simulink model "harness"  (Simulink 7.0)
settings: Solver=ode23  StartTime=0.0  StopTime=20  FixedStep=0.01  RelTol=1e-3
InitFcn:
  | init_simulation
StopFcn:
  | post_simulation
values from neighbouring files (symbols this model uses):
  A = pi*R^2    (= 0.0506707479097)    [constants.m]
  accel_noise = noise_on*.01^2    [constants.m]
  Alpha = pi/180*[-85:5:85]    [constants.m]
  att_noise = noise_on*(.25*pi/180)^2    [constants.m]
  att_ref = [0.2 0.2 0 0 0 0]'    [run_simulation.m]
  att_traj_on = 0    [set_scenario.m]
  b = 0.1    [constants.m]
  const_wind = [1 1 0]    [run_simulation.m]
  g = [0 0 9.8]'    [constants.m]
  gyro_noise = noise_on*.01^2    [constants.m]
  J = [Jxx 0 0 ... (first row only)    [constants.m]
  K_a1s = .009    (= 0.009)    [constants.m]
  K_attitude = [  0   kp_p   kp_y     0    kd_p   kd_y ... (first row only)    [run_simulation.m]
  K_beta = 0.23    [constants.m]
  K_dz = 0.7    [run_simulation.m]
  K_flap = 4*(K_beta + T_nom*dz)*K_a1s/(2*dx)    (= 0.0320793572835)    [constants.m]
  K_pz = .37    (= 0.37)    [run_simulation.m]
  K_torque = 0.47    [constants.m]
  M = 1.8263    [constants.m]
  motor_noise = noise_on*(9.8/4*.05)^2    [constants.m]
  plant_int_period = t_s / tau_motor    (= 0.00131578947368)    [constants.m]
  pos_noise = noise_on*0.02^2    [constants.m]
  r1 = [dx 0 -dz]'    [constants.m]
  r2 = [0 dx -dz]'    [constants.m]
  r3 = [-dx 0 -dz]'    [constants.m]
  r4 = [0 -dx -dz]'    [constants.m]
  R_90 = [0 -1 0 ... (first row only)    [constants.m]
  rho = 1.2    [constants.m]
  select = 0    [run_simulation.m]
  T_nom = M*9.8/4    (= 4.474435)    [constants.m]
  t_s = 1/76    (= 0.0131578947368)    [constants.m]
  tau_motor = 10    [constants.m]
  thrust_max = 9.8 * 1    (= 9.8)    [constants.m]
  thrust_min = 0    [constants.m]
  v_min = 1e-3    (= 0.001)    [constants.m]
  vel_noise = noise_on*0.05^2    [constants.m]
  Vh = sqrt(T/(2*rho*A))    [constants.m]
  Vinf = [0:0.5:6]    [constants.m]
  w_seed = 0    [run_simulation.m]
  wind = 3    [run_simulation.m]
  wind_clip = wind_max    (= 10)    [run_simulation.m]
  wind_duration = 5    [run_simulation.m]
  wind_max = 10    [run_simulation.m]
  wind_start = 3    [run_simulation.m]
  wind_var = (wind_max / 10)^2    (= 1)    [run_simulation.m]
  wind_vector = [1 0 0]'    [run_simulation.m]
  zd_ref = 0    [run_simulation.m]
undefined symbols (not defined in the file or in its folder): DiscIntNeverNeededParam, ToverTh
libraries: simulink x20
(part 2 of 3)

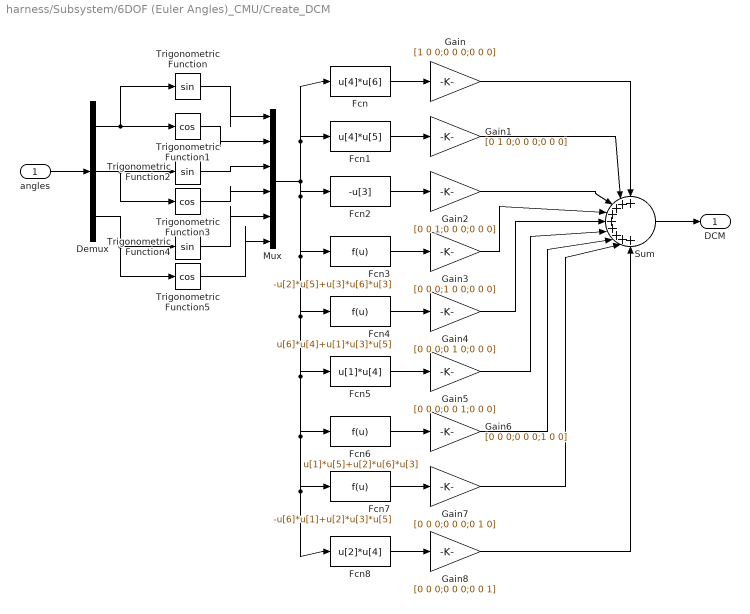
== system harness/Subsystem/6DOF (Euler Angles)_CMU/Create_DCM ==
  angles : Inport  OutDataType=sfix(16)  OutScaling=2^0
  Demux : Demux  Outputs=3
  Fcn : Fcn  Expr=u[4]*u[6]
  Fcn1 : Fcn  Expr=u[4]*u[5]
  Fcn2 : Fcn  Expr=-u[3]
  Fcn3 : Fcn  Expr=-u[2]*u[5]+u[3]*u[6]*u[3]
  Fcn4 : Fcn  Expr=u[6]*u[4]+u[1]*u[3]*u[5]
  Fcn5 : Fcn  Expr=u[1]*u[4]
  Fcn6 : Fcn  Expr=u[1]*u[5]+u[2]*u[6]*u[3]
  Fcn7 : Fcn  Expr=-u[6]*u[1]+u[2]*u[3]*u[5]
  Fcn8 : Fcn  Expr=u[2]*u[4]
  Gain : Gain  Gain=[1 0 0;0 0 0;0 0 0]  ParameterDataType=sfix(16)  ParameterScaling=2^0  OutDataType=sfix(16)  OutScaling=2^0
  Gain1 : Gain  Gain=[0 1 0;0 0 0;0 0 0]  ParameterDataType=sfix(16)  ParameterScaling=2^0  OutDataType=sfix(16)  OutScaling=2^0
  Gain2 : Gain  Gain=[0 0 1;0 0 0;0 0 0]  ParameterDataType=sfix(16)  ParameterScaling=2^0  OutDataType=sfix(16)  OutScaling=2^0
  Gain3 : Gain  Gain=[0 0 0;1 0 0;0 0 0]  ParameterDataType=sfix(16)  ParameterScaling=2^0  OutDataType=sfix(16)  OutScaling=2^0
  Gain4 : Gain  Gain=[0 0 0;0 1 0;0 0 0]  ParameterDataType=sfix(16)  ParameterScaling=2^0  OutDataType=sfix(16)  OutScaling=2^0
  Gain5 : Gain  Gain=[0 0 0;0 0 1;0 0 0]  ParameterDataType=sfix(16)  ParameterScaling=2^0  OutDataType=sfix(16)  OutScaling=2^0
  Gain6 : Gain  Gain=[0 0 0;0 0 0;1 0 0]  ParameterDataType=sfix(16)  ParameterScaling=2^0  OutDataType=sfix(16)  OutScaling=2^0
  Gain7 : Gain  Gain=[0 0 0;0 0 0;0 1 0]  ParameterDataType=sfix(16)  ParameterScaling=2^0  OutDataType=sfix(16)  OutScaling=2^0
  Gain8 : Gain  Gain=[0 0 0;0 0 0;0 0 1]  ParameterDataType=sfix(16)  ParameterScaling=2^0  OutDataType=sfix(16)  OutScaling=2^0
  Mux : Mux  Inputs=6
  Sum : Sum  Inputs=+++++++++  OutDataType=sfix(16)  OutScaling=2^0
  Trigonometric Function : Trigonometry
  Trigonometric Function1 : Trigonometry  Operator=cos
  Trigonometric Function2 : Trigonometry
  Trigonometric Function3 : Trigonometry  Operator=cos
  Trigonometric Function4 : Trigonometry
  Trigonometric Function5 : Trigonometry  Operator=cos
  DCM : Outport  OutDataType=sfix(16)  OutScaling=2^0
  wires:
  Sum/1 -> DCM/1
  Gain8/1 -> Sum/9
  Fcn8/1 -> Gain8/1
  Gain7/1 -> Sum/8
  Fcn7/1 -> Gain7/1
  Gain6/1 -> Sum/7
  Fcn6/1 -> Gain6/1
  Gain5/1 -> Sum/6
  Fcn5/1 -> Gain5/1
  Gain4/1 -> Sum/5
  Fcn4/1 -> Gain4/1
  Gain3/1 -> Sum/4
  Fcn3/1 -> Gain3/1
  Gain2/1 -> Sum/3
  Fcn2/1 -> Gain2/1
  Gain1/1 -> Sum/2
  Fcn1/1 -> Gain1/1
  Gain/1 -> Sum/1
  Fcn/1 -> Gain/1
  Mux/1 -> Fcn8/1, Fcn7/1, Fcn6/1, Fcn5/1, Fcn4/1, Fcn3/1, Fcn2/1, Fcn1/1, Fcn/1
  Trigonometric Function5/1 -> Mux/6
  Trigonometric Function4/1 -> Mux/5
  Trigonometric Function3/1 -> Mux/4
  Trigonometric Function2/1 -> Mux/3
  Trigonometric Function1/1 -> Mux/2
  Trigonometric Function/1 -> Mux/1
  Demux/3 -> Trigonometric Function5/1, Trigonometric Function4/1
  Demux/2 -> Trigonometric Function3/1, Trigonometric Function2/1
  Demux/1 -> Trigonometric Function1/1, Trigonometric Function/1
  angles/1 -> Demux/1

== system harness/Subsystem/6DOF (Euler Angles)_CMU/CrossProduct(AXB) ==
  A : Inport  OutDataType=sfix(16)  OutScaling=2^0
  B : Inport  Port=2  OutDataType=sfix(16)  OutScaling=2^0
  Fcn : Fcn  Expr=u[2]*u[6]-u[3]*u[5]
  Fcn1 : Fcn  Expr=u[3]*u[4]-u[1]*u[6]
  Fcn2 : Fcn  Expr=u[1]*u[5]-u[2]*u[4]
  Mux : Mux  Inputs=2
  Mux1 : Mux  Inputs=3
  Out : Outport  OutDataType=sfix(16)  OutScaling=2^0
  wires:
  Mux1/1 -> Out/1
  Fcn2/1 -> Mux1/3
  Fcn1/1 -> Mux1/2
  Fcn/1 -> Mux1/1
  Mux/1 -> Fcn2/1, Fcn1/1, Fcn/1
  B/1 -> Mux/2
  A/1 -> Mux/1

== system harness/Subsystem/6DOF (Euler Angles)_CMU/CrossProduct(AXB)1 ==
  A : Inport  OutDataType=sfix(16)  OutScaling=2^0
  B : Inport  Port=2  OutDataType=sfix(16)  OutScaling=2^0
  Fcn : Fcn  Expr=u[2]*u[6]-u[3]*u[5]
  Fcn1 : Fcn  Expr=u[3]*u[4]-u[1]*u[6]
  Fcn2 : Fcn  Expr=u[1]*u[5]-u[2]*u[4]
  Mux : Mux  Inputs=2
  Mux1 : Mux  Inputs=3
  Out : Outport  OutDataType=sfix(16)  OutScaling=2^0
  wires:
  A/1 -> Mux/1
  B/1 -> Mux/2
  Mux/1 -> Fcn/1, Fcn1/1, Fcn2/1
  Fcn/1 -> Mux1/1
  Fcn1/1 -> Mux1/2
  Fcn2/1 -> Mux1/3
  Mux1/1 -> Out/1

== system harness/Subsystem/Aerodynamic Effects/Flapping Dynamics ==
  Vb2_hat : Inport  OutDataType=sfix(16)  OutScaling=2^0
  "Body Z " : Constant  Value=[0; 0; -1];  OutDataType=sfix(16)  OutScaling=2^0
  Constant : Constant  OutDataType=sfix(16)  OutScaling=2^0
  Constant1 : Constant  Value=1/v_min  OutDataType=sfix(16)  OutScaling=2^0
  Constant2 : Constant  Value=[0 0 0]'  OutDataType=sfix(16)  OutScaling=2^0
  Divide : Product  Inputs=*/  OutDataType=sfix(16)  OutScaling=2^-10
  Dot Product : simulink/Math Operations/Dot Product  InputSameDT=on  OutDataType=sfix(16)  OutScaling=2^-10  DoSatur=off
  Flap Angle Gain : Gain  Gain=K_a1s  ParameterDataType=sfix(16)  ParameterScaling=2^0  OutDataType=sfix(16)  OutScaling=2^0
  Gain : Gain  Gain=-1  ParameterDataType=sfix(16)  ParameterScaling=2^0  OutDataType=sfix(16)  OutScaling=2^0
  Gain1 : Gain  Gain=K_beta  ParameterDataType=sfix(16)  ParameterScaling=2^0  OutDataType=sfix(16)  OutScaling=2^0
  Gain2 : Gain  Gain=4  ParameterDataType=sfix(16)  ParameterScaling=2^0  OutDataType=sfix(16)  OutScaling=2^0
  Math Function : Math  Operator=sqrt  OutDataType=sfix(16)  OutScaling=2^0  SaturateOnIntegerOverflow=on
  Product{1..4} (4 alike) : Product  OutDataType=sfix(16)  OutScaling=2^0  RndMeth=Zero
  Sum : Sum  Inputs=|++  OutDataType=sfix(16)  OutScaling=2^0
  Switch : Switch  Threshold=v_min
  Trigonometric Function : Trigonometry
  Trigonometric Function1 : Trigonometry  Operator=cos
  flap moments : Scope
      settings: SaveName=ScopeData10
  flapping switch : Switch  Threshold=v_min
  rotate 90 degrees : Gain  Gain=R_90  Multiplication=Matrix(K*u)  ParameterDataType=sfix(16)  ParameterScaling=2^0  OutDataType=sfix(16)  OutScaling=2^0
  v : Scope
      settings: SaveName=ScopeData6
  thrust vector : Outport  OutDataType=sfix(16)  OutScaling=2^0
  rotor blade moments : Outport  Port=2  OutDataType=sfix(16)  OutScaling=2^0
  wires:
  Product4/1 -> Trigonometric Function1/1, Trigonometric Function/1, Gain1/1, v/1  "flap angle"
  Vb2_hat/1 -> Dot Product/1, Dot Product/2, Divide/1
  Dot Product/1 -> Math Function/1
  Math Function/1 -> Switch/1, Switch/2, flapping switch/2, Flap Angle Gain/1  "v"
  Trigonometric Function1/1 -> Product1/2
  Trigonometric Function/1 -> Product3/1
  Product3/1 -> Sum/2
  Gain/1 -> Product3/2
  Product1/1 -> Sum/1
  "Body Z "/1 -> Product1/1
  Sum/1 -> thrust vector/1
  Gain2/1 -> rotor blade moments/1, flap moments/1
  Switch/1 -> Divide/2
  Constant1/1 -> Switch/3
  Divide/1 -> flapping switch/1  "unit vector"
  flapping switch/1 -> Gain/1, rotate 90 degrees/1
  Constant2/1 -> flapping switch/3
  Product2/1 -> Gain2/1
  rotate 90 degrees/1 -> Product2/2
  Gain1/1 -> Product2/1
  Flap Angle Gain/1 -> Product4/2
  Constant/1 -> Product4/1

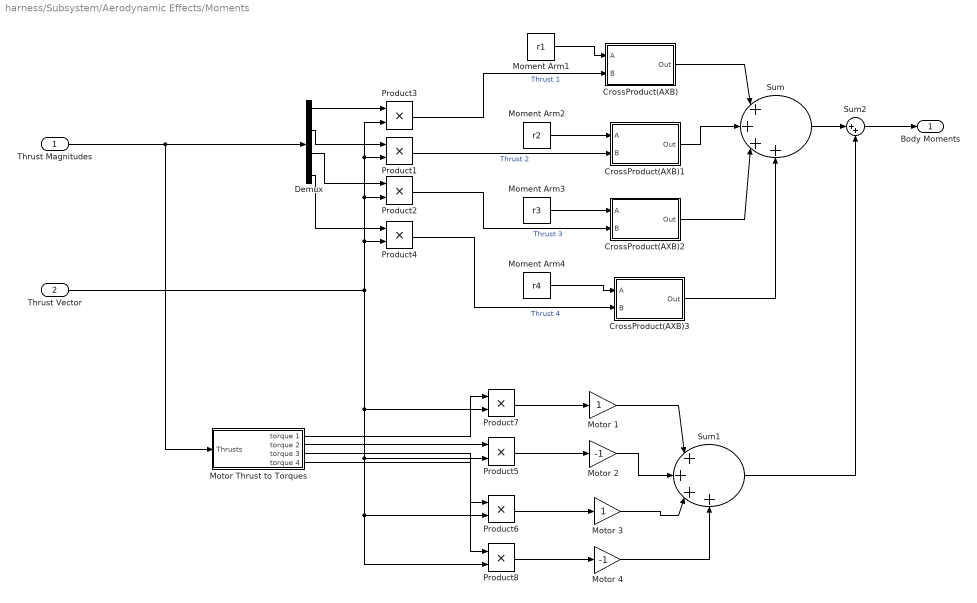
== system harness/Subsystem/Aerodynamic Effects/Moments ==
  Thrust Magnitudes : Inport  OutDataType=sfix(16)  OutScaling=2^0
  Thrust Vector : Inport  Port=2  OutDataType=sfix(16)  OutScaling=2^0
  CrossProduct(AXB) : Subsystem
  CrossProduct(AXB)1 : Subsystem
  CrossProduct(AXB)2 : Subsystem
  CrossProduct(AXB)3 : Subsystem
  Demux : Demux
  Moment Arm1 : Constant  Value=r1  OutDataType=sfix(16)  OutScaling=2^0
  Moment Arm2 : Constant  Value=r2  OutDataType=sfix(16)  OutScaling=2^0
  Moment Arm3 : Constant  Value=r3  OutDataType=sfix(16)  OutScaling=2^0
  Moment Arm4 : Constant  Value=r4  OutDataType=sfix(16)  OutScaling=2^0
  Motor 1 : Gain  ParameterDataType=sfix(16)  ParameterScaling=2^0  OutDataType=sfix(16)  OutScaling=2^0
  Motor 2 : Gain  Gain=-1  ParameterDataType=sfix(16)  ParameterScaling=2^0  OutDataType=sfix(16)  OutScaling=2^0
  Motor 3 : Gain  ParameterDataType=sfix(16)  ParameterScaling=2^0  OutDataType=sfix(16)  OutScaling=2^0
  Motor 4 : Gain  Gain=-1  ParameterDataType=sfix(16)  ParameterScaling=2^0  OutDataType=sfix(16)  OutScaling=2^0
  Motor Thrust to Torques : Subsystem
  Product{1..8} (8 alike) : Product  OutDataType=sfix(16)  OutScaling=2^0  RndMeth=Zero
  Sum : Sum  Inputs=|++++  OutDataType=sfix(16)  OutScaling=2^0
  Sum1 : Sum  Inputs=|++++  OutDataType=sfix(16)  OutScaling=2^0
  Sum2 : Sum  Inputs=|++  OutDataType=sfix(16)  OutScaling=2^0
  Body Moments : Outport  OutDataType=sfix(16)  OutScaling=2^0
  wires:
  Thrust Magnitudes/1 -> Demux/1, Motor Thrust to Torques/1(Thrusts)
  Demux/1 -> Product3/1
  Demux/2 -> Product1/1
  Demux/3 -> Product2/1
  Demux/4 -> Product4/1
  Thrust Vector/1 -> Product3/2, Product1/2, Product2/2, Product4/2, Product7/2, Product5/2, Product6/2, Product8/2
  Moment Arm1/1 -> CrossProduct(AXB)/1(A)
  Product3/1 -> CrossProduct(AXB)/2(B)  "Thrust 1"
  Moment Arm2/1 -> CrossProduct(AXB)1/1(A)
  Product1/1 -> CrossProduct(AXB)1/2(B)  "Thrust 2"
  Moment Arm3/1 -> CrossProduct(AXB)2/1(A)
  Product2/1 -> CrossProduct(AXB)2/2(B)  "Thrust 3"
  Moment Arm4/1 -> CrossProduct(AXB)3/1(A)
  Product4/1 -> CrossProduct(AXB)3/2(B)  "Thrust 4"
  CrossProduct(AXB)/1(Out) -> Sum/1
  CrossProduct(AXB)2/1(Out) -> Sum/3
  CrossProduct(AXB)3/1(Out) -> Sum/4
  Motor 1/1 -> Sum1/1
  Motor 2/1 -> Sum1/2
  Motor 3/1 -> Sum1/3
  Motor 4/1 -> Sum1/4
  Sum/1 -> Sum2/1
  Sum1/1 -> Sum2/2
  Sum2/1 -> Body Moments/1
  Product7/1 -> Motor 1/1
  Product5/1 -> Motor 2/1
  Product6/1 -> Motor 3/1
  Product8/1 -> Motor 4/1
  Motor Thrust to Torques/1(torque 1) -> Product7/1
  Motor Thrust to Torques/2(torque 2) -> Product5/1
  Motor Thrust to Torques/3(torque 3) -> Product6/1
  Motor Thrust to Torques/4(torque 4) -> Product8/1
  CrossProduct(AXB)1/1(Out) -> Sum/2

== system harness/Subsystem/Aerodynamic Effects/Vertical Effect Dynamics ==
  Thrust Command : Inport  OutDataType=sfix(16)  OutScaling=2^0
  V (body) : Inport  Port=2  OutDataType=sfix(16)  OutScaling=2^0
  Demux : Demux
  Motor 1 Vertical Effect Dynamics : Subsystem
  Motor 2 Vertical Effect Dynamics : Subsystem
  Motor 3 Vertical Effect Dynamics : Subsystem
  Motor 4 Vertical Effect Dynamics : Subsystem
  Mux : Mux
  Saturation{1..4} (4 alike) : Saturate  UpperLimit=2  LowerLimit=0.5
  Thrust Multipliers : Scope
      settings: YMin=0.975  YMax=1.225  SaveName=ScopeData14
  Zero-Order Hold : ZeroOrderHold  SampleTime=1/tau_motor
  Zero-Order Hold1 : ZeroOrderHold  SampleTime=1/tau_motor
  Thrust Multiplier : Outport  OutDataType=sfix(16)  OutScaling=2^0
  wires:
  Thrust Command/1 -> Zero-Order Hold1/1
  Mux/1 -> Thrust Multiplier/1, Thrust Multipliers/1
  Demux/1 -> Motor 1 Vertical Effect Dynamics/1(Thrust Command)
  Demux/2 -> Motor 2 Vertical Effect Dynamics/1(Thrust Command)
  Demux/3 -> Motor 3 Vertical Effect Dynamics/1(Thrust Command)
  Demux/4 -> Motor 4 Vertical Effect Dynamics/1(Thrust Command)
  Motor 1 Vertical Effect Dynamics/1(Thrust Multiplier) -> Saturation1/1
  Motor 2 Vertical Effect Dynamics/1(Thrust Multiplier) -> Saturation2/1
  Motor 3 Vertical Effect Dynamics/1(Thrust Multiplier) -> Saturation3/1
  Motor 4 Vertical Effect Dynamics/1(Thrust Multiplier) -> Saturation4/1
  Saturation1/1 -> Mux/1
  Saturation2/1 -> Mux/2
  Saturation3/1 -> Mux/3
  Saturation4/1 -> Mux/4
  V (body)/1 -> Zero-Order Hold/1
  Zero-Order Hold/1 -> Motor 1 Vertical Effect Dynamics/2(V (body)), Motor 2 Vertical Effect Dynamics/2(V (body)), Motor 3 Vertical Effect Dynamics/2(V (body)), Motor 4 Vertical Effect Dynamics/2(V (body))
  Zero-Order Hold1/1 -> Demux/1

== system harness/Subsystem/Motor Dynamics/Motor Noise Source ==
  Motor Noise : RandomNumber  Variance=motor_noise  SampleTime=t_s
  Motor Noise1 : RandomNumber  Variance=motor_noise  Seed=1  SampleTime=t_s
  Motor Noise2 : RandomNumber  Variance=motor_noise  Seed=2  SampleTime=t_s
  Motor Noise3 : RandomNumber  Variance=motor_noise  Seed=3  SampleTime=t_s
  Motor 1 : Outport  OutDataType=sfix(16)  OutScaling=2^0
  Motor 2 : Outport  Port=2  OutDataType=sfix(16)  OutScaling=2^0
  Motor 3 : Outport  Port=3  OutDataType=sfix(16)  OutScaling=2^0
  Motor 4 : Outport  Port=4  OutDataType=sfix(16)  OutScaling=2^0
  wires:
  Motor Noise/1 -> Motor 1/1
  Motor Noise1/1 -> Motor 2/1
  Motor Noise2/1 -> Motor 3/1
  Motor Noise3/1 -> Motor 4/1

== system harness/Subsystem1/6DOF (Euler Angles)_CMU/Body-based-to-ref-frame-based ==
  note: dF/dt = P + Q sinF tanQ + R cosF tanQ
      | dQ/dt = Q cosF - R sinF
      | dY/dt = Q sinF secQ + R cosF secQ
  omega : Inport  OutDataType=sfix(16)  OutScaling=2^0
  theta : Inport  Port=2  OutDataType=sfix(16)  OutScaling=2^0
  Fcn : Fcn  Expr=u[1]+u[2]*sin(u[4])*tan(u[5])+u[3]*cos(u[4])*tan(u[5])
  Fcn1 : Fcn  Expr=u[2]*cos(u[4])-u[3]*sin(u[4])
  Fcn2 : Fcn  Expr=u[2]*sin(u[4])*(1/cos(u[5]))+u[3]*cos(u[4])*(1/cos(u[5]))
  Mux : Mux  Inputs=2
  Mux1 : Mux  Inputs=3
  Out1 : Outport  OutDataType=sfix(16)  OutScaling=2^0
  wires:
  Mux1/1 -> Out1/1
  Fcn2/1 -> Mux1/3
  Fcn1/1 -> Mux1/2
  Fcn/1 -> Mux1/1
  Mux/1 -> Fcn2/1, Fcn1/1, Fcn/1
  theta/1 -> Mux/2
  omega/1 -> Mux/1

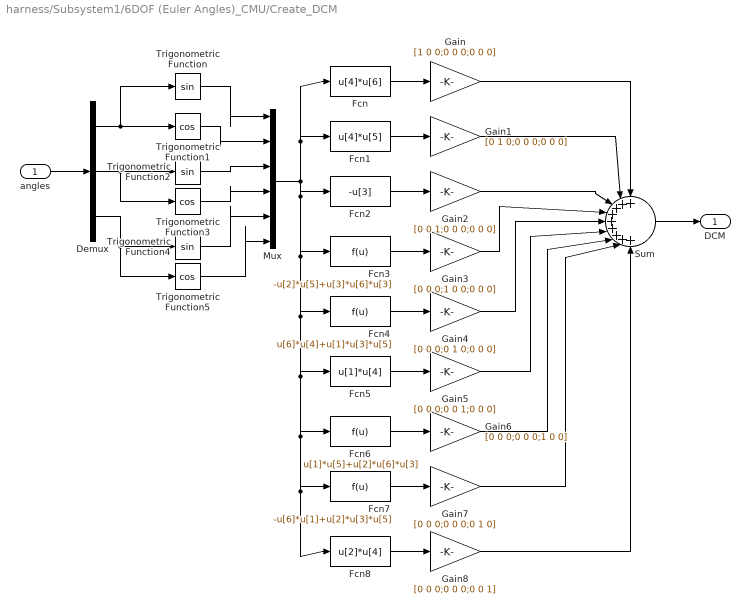
== system harness/Subsystem1/6DOF (Euler Angles)_CMU/Create_DCM ==
  angles : Inport  OutDataType=sfix(16)  OutScaling=2^0
  Demux : Demux  Outputs=3
  Fcn : Fcn  Expr=u[4]*u[6]
  Fcn1 : Fcn  Expr=u[4]*u[5]
  Fcn2 : Fcn  Expr=-u[3]
  Fcn3 : Fcn  Expr=-u[2]*u[5]+u[3]*u[6]*u[3]
  Fcn4 : Fcn  Expr=u[6]*u[4]+u[1]*u[3]*u[5]
  Fcn5 : Fcn  Expr=u[1]*u[4]
  Fcn6 : Fcn  Expr=u[1]*u[5]+u[2]*u[6]*u[3]
  Fcn7 : Fcn  Expr=-u[6]*u[1]+u[2]*u[3]*u[5]
  Fcn8 : Fcn  Expr=u[2]*u[4]
  Gain : Gain  Gain=[1 0 0;0 0 0;0 0 0]  ParameterDataType=sfix(16)  ParameterScaling=2^0  OutDataType=sfix(16)  OutScaling=2^0
  Gain1 : Gain  Gain=[0 1 0;0 0 0;0 0 0]  ParameterDataType=sfix(16)  ParameterScaling=2^0  OutDataType=sfix(16)  OutScaling=2^0
  Gain2 : Gain  Gain=[0 0 1;0 0 0;0 0 0]  ParameterDataType=sfix(16)  ParameterScaling=2^0  OutDataType=sfix(16)  OutScaling=2^0
  Gain3 : Gain  Gain=[0 0 0;1 0 0;0 0 0]  ParameterDataType=sfix(16)  ParameterScaling=2^0  OutDataType=sfix(16)  OutScaling=2^0
  Gain4 : Gain  Gain=[0 0 0;0 1 0;0 0 0]  ParameterDataType=sfix(16)  ParameterScaling=2^0  OutDataType=sfix(16)  OutScaling=2^0
  Gain5 : Gain  Gain=[0 0 0;0 0 1;0 0 0]  ParameterDataType=sfix(16)  ParameterScaling=2^0  OutDataType=sfix(16)  OutScaling=2^0
  Gain6 : Gain  Gain=[0 0 0;0 0 0;1 0 0]  ParameterDataType=sfix(16)  ParameterScaling=2^0  OutDataType=sfix(16)  OutScaling=2^0
  Gain7 : Gain  Gain=[0 0 0;0 0 0;0 1 0]  ParameterDataType=sfix(16)  ParameterScaling=2^0  OutDataType=sfix(16)  OutScaling=2^0
  Gain8 : Gain  Gain=[0 0 0;0 0 0;0 0 1]  ParameterDataType=sfix(16)  ParameterScaling=2^0  OutDataType=sfix(16)  OutScaling=2^0
  Mux : Mux  Inputs=6
  Sum : Sum  Inputs=+++++++++  OutDataType=sfix(16)  OutScaling=2^0
  Trigonometric Function : Trigonometry
  Trigonometric Function1 : Trigonometry  Operator=cos
  Trigonometric Function2 : Trigonometry
  Trigonometric Function3 : Trigonometry  Operator=cos
  Trigonometric Function4 : Trigonometry
  Trigonometric Function5 : Trigonometry  Operator=cos
  DCM : Outport  OutDataType=sfix(16)  OutScaling=2^0
  wires:
  Sum/1 -> DCM/1
  Gain8/1 -> Sum/9
  Fcn8/1 -> Gain8/1
  Gain7/1 -> Sum/8
  Fcn7/1 -> Gain7/1
  Gain6/1 -> Sum/7
  Fcn6/1 -> Gain6/1
  Gain5/1 -> Sum/6
  Fcn5/1 -> Gain5/1
  Gain4/1 -> Sum/5
  Fcn4/1 -> Gain4/1
  Gain3/1 -> Sum/4
  Fcn3/1 -> Gain3/1
  Gain2/1 -> Sum/3
  Fcn2/1 -> Gain2/1
  Gain1/1 -> Sum/2
  Fcn1/1 -> Gain1/1
  Gain/1 -> Sum/1
  Fcn/1 -> Gain/1
  Mux/1 -> Fcn8/1, Fcn7/1, Fcn6/1, Fcn5/1, Fcn4/1, Fcn3/1, Fcn2/1, Fcn1/1, Fcn/1
  Trigonometric Function5/1 -> Mux/6
  Trigonometric Function4/1 -> Mux/5
  Trigonometric Function3/1 -> Mux/4
  Trigonometric Function2/1 -> Mux/3
  Trigonometric Function1/1 -> Mux/2
  Trigonometric Function/1 -> Mux/1
  Demux/3 -> Trigonometric Function5/1, Trigonometric Function4/1
  Demux/2 -> Trigonometric Function3/1, Trigonometric Function2/1
  Demux/1 -> Trigonometric Function1/1, Trigonometric Function/1
  angles/1 -> Demux/1

== system harness/Subsystem1/6DOF (Euler Angles)_CMU/CrossProduct(AXB) ==
  A : Inport  OutDataType=sfix(16)  OutScaling=2^0
  B : Inport  Port=2  OutDataType=sfix(16)  OutScaling=2^0
  Fcn : Fcn  Expr=u[2]*u[6]-u[3]*u[5]
  Fcn1 : Fcn  Expr=u[3]*u[4]-u[1]*u[6]
  Fcn2 : Fcn  Expr=u[1]*u[5]-u[2]*u[4]
  Mux : Mux  Inputs=2
  Mux1 : Mux  Inputs=3
  Out : Outport  OutDataType=sfix(16)  OutScaling=2^0
  wires:
  Mux1/1 -> Out/1
  Fcn2/1 -> Mux1/3
  Fcn1/1 -> Mux1/2
  Fcn/1 -> Mux1/1
  Mux/1 -> Fcn2/1, Fcn1/1, Fcn/1
  B/1 -> Mux/2
  A/1 -> Mux/1

== system harness/Subsystem1/6DOF (Euler Angles)_CMU/CrossProduct(AXB)1 ==
  A : Inport  OutDataType=sfix(16)  OutScaling=2^0
  B : Inport  Port=2  OutDataType=sfix(16)  OutScaling=2^0
  Fcn : Fcn  Expr=u[2]*u[6]-u[3]*u[5]
  Fcn1 : Fcn  Expr=u[3]*u[4]-u[1]*u[6]
  Fcn2 : Fcn  Expr=u[1]*u[5]-u[2]*u[4]
  Mux : Mux  Inputs=2
  Mux1 : Mux  Inputs=3
  Out : Outport  OutDataType=sfix(16)  OutScaling=2^0
  wires:
  A/1 -> Mux/1
  B/1 -> Mux/2
  Mux/1 -> Fcn/1, Fcn1/1, Fcn2/1
  Fcn/1 -> Mux1/1
  Fcn1/1 -> Mux1/2
  Fcn2/1 -> Mux1/3
  Mux1/1 -> Out/1

== system harness/Subsystem1/Aerodynamic Effects/Flapping Dynamics ==
  Vb2_hat : Inport  OutDataType=sfix(16)  OutScaling=2^0
  "Body Z " : Constant  Value=[0; 0; -1];  OutDataType=sfix(16)  OutScaling=2^0
  Constant : Constant  OutDataType=sfix(16)  OutScaling=2^0
  Constant1 : Constant  Value=1/v_min  OutDataType=sfix(16)  OutScaling=2^0
  Constant2 : Constant  Value=[0 0 0]'  OutDataType=sfix(16)  OutScaling=2^0
  Divide : Product  Inputs=*/  OutDataType=sfix(16)  OutScaling=2^-10
  Dot Product : simulink/Math Operations/Dot Product  InputSameDT=on  OutDataType=sfix(16)  OutScaling=2^-10  DoSatur=off
  Flap Angle Gain : Gain  Gain=K_a1s  ParameterDataType=sfix(16)  ParameterScaling=2^0  OutDataType=sfix(16)  OutScaling=2^0
  Gain : Gain  Gain=-1  ParameterDataType=sfix(16)  ParameterScaling=2^0  OutDataType=sfix(16)  OutScaling=2^0
  Gain1 : Gain  Gain=K_beta  ParameterDataType=sfix(16)  ParameterScaling=2^0  OutDataType=sfix(16)  OutScaling=2^0
  Gain2 : Gain  Gain=4  ParameterDataType=sfix(16)  ParameterScaling=2^0  OutDataType=sfix(16)  OutScaling=2^0
  Math Function : Math  Operator=sqrt  OutDataType=sfix(16)  OutScaling=2^0  SaturateOnIntegerOverflow=on
  Product{1..4} (4 alike) : Product  OutDataType=sfix(16)  OutScaling=2^0  RndMeth=Zero
  Sum : Sum  Inputs=|++  OutDataType=sfix(16)  OutScaling=2^0
  Switch : Switch  Threshold=v_min
  Trigonometric Function : Trigonometry
  Trigonometric Function1 : Trigonometry  Operator=cos
  flap moments : Scope
      settings: SaveName=ScopeData10
  flapping switch : Switch  Threshold=v_min
  rotate 90 degrees : Gain  Gain=R_90  Multiplication=Matrix(K*u)  ParameterDataType=sfix(16)  ParameterScaling=2^0  OutDataType=sfix(16)  OutScaling=2^0
  v : Scope
      settings: SaveName=ScopeData6
  thrust vector : Outport  OutDataType=sfix(16)  OutScaling=2^0
  rotor blade moments : Outport  Port=2  OutDataType=sfix(16)  OutScaling=2^0
  wires:
  Product4/1 -> Trigonometric Function1/1, Trigonometric Function/1, Gain1/1, v/1  "flap angle"
  Vb2_hat/1 -> Dot Product/1, Dot Product/2, Divide/1
  Dot Product/1 -> Math Function/1
  Math Function/1 -> Switch/1, Switch/2, flapping switch/2, Flap Angle Gain/1  "v"
  Trigonometric Function1/1 -> Product1/2
  Trigonometric Function/1 -> Product3/1
  Product3/1 -> Sum/2
  Gain/1 -> Product3/2
  Product1/1 -> Sum/1
  "Body Z "/1 -> Product1/1
  Sum/1 -> thrust vector/1
  Gain2/1 -> rotor blade moments/1, flap moments/1
  Switch/1 -> Divide/2
  Constant1/1 -> Switch/3
  Divide/1 -> flapping switch/1  "unit vector"
  flapping switch/1 -> Gain/1, rotate 90 degrees/1
  Constant2/1 -> flapping switch/3
  Product2/1 -> Gain2/1
  rotate 90 degrees/1 -> Product2/2
  Gain1/1 -> Product2/1
  Flap Angle Gain/1 -> Product4/2
  Constant/1 -> Product4/1

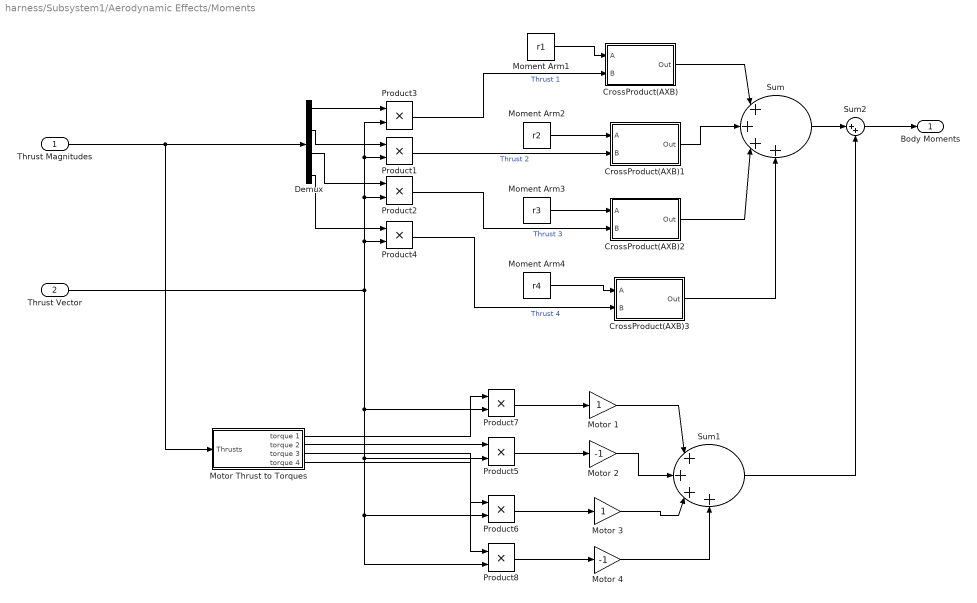
== system harness/Subsystem1/Aerodynamic Effects/Moments ==
  Thrust Magnitudes : Inport  OutDataType=sfix(16)  OutScaling=2^0
  Thrust Vector : Inport  Port=2  OutDataType=sfix(16)  OutScaling=2^0
  CrossProduct(AXB) : Subsystem
  CrossProduct(AXB)1 : Subsystem
  CrossProduct(AXB)2 : Subsystem
  CrossProduct(AXB)3 : Subsystem
  Demux : Demux
  Moment Arm1 : Constant  Value=r1  OutDataType=sfix(16)  OutScaling=2^0
  Moment Arm2 : Constant  Value=r2  OutDataType=sfix(16)  OutScaling=2^0
  Moment Arm3 : Constant  Value=r3  OutDataType=sfix(16)  OutScaling=2^0
  Moment Arm4 : Constant  Value=r4  OutDataType=sfix(16)  OutScaling=2^0
  Motor 1 : Gain  ParameterDataType=sfix(16)  ParameterScaling=2^0  OutDataType=sfix(16)  OutScaling=2^0
  Motor 2 : Gain  Gain=-1  ParameterDataType=sfix(16)  ParameterScaling=2^0  OutDataType=sfix(16)  OutScaling=2^0
  Motor 3 : Gain  ParameterDataType=sfix(16)  ParameterScaling=2^0  OutDataType=sfix(16)  OutScaling=2^0
  Motor 4 : Gain  Gain=-1  ParameterDataType=sfix(16)  ParameterScaling=2^0  OutDataType=sfix(16)  OutScaling=2^0
  Motor Thrust to Torques : Subsystem
  Product{1..8} (8 alike) : Product  OutDataType=sfix(16)  OutScaling=2^0  RndMeth=Zero
  Sum : Sum  Inputs=|++++  OutDataType=sfix(16)  OutScaling=2^0
  Sum1 : Sum  Inputs=|++++  OutDataType=sfix(16)  OutScaling=2^0
  Sum2 : Sum  Inputs=|++  OutDataType=sfix(16)  OutScaling=2^0
  Body Moments : Outport  OutDataType=sfix(16)  OutScaling=2^0
  wires:
  Thrust Magnitudes/1 -> Demux/1, Motor Thrust to Torques/1(Thrusts)
  Demux/1 -> Product3/1
  Demux/2 -> Product1/1
  Demux/3 -> Product2/1
  Demux/4 -> Product4/1
  Thrust Vector/1 -> Product3/2, Product1/2, Product2/2, Product4/2, Product7/2, Product5/2, Product6/2, Product8/2
  Moment Arm1/1 -> CrossProduct(AXB)/1(A)
  Product3/1 -> CrossProduct(AXB)/2(B)  "Thrust 1"
  Moment Arm2/1 -> CrossProduct(AXB)1/1(A)
  Product1/1 -> CrossProduct(AXB)1/2(B)  "Thrust 2"
  Moment Arm3/1 -> CrossProduct(AXB)2/1(A)
  Product2/1 -> CrossProduct(AXB)2/2(B)  "Thrust 3"
  Moment Arm4/1 -> CrossProduct(AXB)3/1(A)
  Product4/1 -> CrossProduct(AXB)3/2(B)  "Thrust 4"
  CrossProduct(AXB)/1(Out) -> Sum/1
  CrossProduct(AXB)2/1(Out) -> Sum/3
  CrossProduct(AXB)3/1(Out) -> Sum/4
  Motor 1/1 -> Sum1/1
  Motor 2/1 -> Sum1/2
  Motor 3/1 -> Sum1/3
  Motor 4/1 -> Sum1/4
  Sum/1 -> Sum2/1
  Sum1/1 -> Sum2/2
  Sum2/1 -> Body Moments/1
  Product7/1 -> Motor 1/1
  Product5/1 -> Motor 2/1
  Product6/1 -> Motor 3/1
  Product8/1 -> Motor 4/1
  Motor Thrust to Torques/1(torque 1) -> Product7/1
  Motor Thrust to Torques/2(torque 2) -> Product5/1
  Motor Thrust to Torques/3(torque 3) -> Product6/1
  Motor Thrust to Torques/4(torque 4) -> Product8/1
  CrossProduct(AXB)1/1(Out) -> Sum/2

== system harness/Subsystem1/Aerodynamic Effects/Vertical Effect Dynamics ==
  Thrust Command : Inport  OutDataType=sfix(16)  OutScaling=2^0
  V (body) : Inport  Port=2  OutDataType=sfix(16)  OutScaling=2^0
  Demux : Demux
  Motor 1 Vertical Effect Dynamics : Subsystem
  Motor 2 Vertical Effect Dynamics : Subsystem
  Motor 3 Vertical Effect Dynamics : Subsystem
  Motor 4 Vertical Effect Dynamics : Subsystem
  Mux : Mux
  Saturation{1..4} (4 alike) : Saturate  UpperLimit=2  LowerLimit=0.5
  Thrust Multipliers : Scope
      settings: YMin=0.975  YMax=1.225  SaveName=ScopeData14
  Zero-Order Hold : ZeroOrderHold  SampleTime=plant_int_period
  Zero-Order Hold1 : ZeroOrderHold  SampleTime=plant_int_period
  Thrust Multiplier : Outport  OutDataType=sfix(16)  OutScaling=2^0
  wires:
  Thrust Command/1 -> Zero-Order Hold1/1
  Mux/1 -> Thrust Multiplier/1, Thrust Multipliers/1
  Demux/1 -> Motor 1 Vertical Effect Dynamics/1(Thrust Command)
  Demux/2 -> Motor 2 Vertical Effect Dynamics/1(Thrust Command)
  Demux/3 -> Motor 3 Vertical Effect Dynamics/1(Thrust Command)
  Demux/4 -> Motor 4 Vertical Effect Dynamics/1(Thrust Command)
  Motor 1 Vertical Effect Dynamics/1(Thrust Multiplier) -> Saturation1/1
  Motor 2 Vertical Effect Dynamics/1(Thrust Multiplier) -> Saturation2/1
  Motor 3 Vertical Effect Dynamics/1(Thrust Multiplier) -> Saturation3/1
  Motor 4 Vertical Effect Dynamics/1(Thrust Multiplier) -> Saturation4/1
  Saturation1/1 -> Mux/1
  Saturation2/1 -> Mux/2
  Saturation3/1 -> Mux/3
  Saturation4/1 -> Mux/4
  V (body)/1 -> Zero-Order Hold/1
  Zero-Order Hold/1 -> Motor 1 Vertical Effect Dynamics/2(V (body)), Motor 2 Vertical Effect Dynamics/2(V (body)), Motor 3 Vertical Effect Dynamics/2(V (body)), Motor 4 Vertical Effect Dynamics/2(V (body))
  Zero-Order Hold1/1 -> Demux/1

== system harness/Subsystem1/Motor Dynamics/Motor Noise Source ==
  Motor Noise : RandomNumber  Variance=motor_noise  SampleTime=plant_int_period
  Motor Noise1 : RandomNumber  Variance=motor_noise  Seed=1  SampleTime=plant_int_period
  Motor Noise2 : RandomNumber  Variance=motor_noise  Seed=2  SampleTime=plant_int_period
  Motor Noise3 : RandomNumber  Variance=motor_noise  Seed=3  SampleTime=plant_int_period
  Motor 1 : Outport  OutDataType=sfix(16)  OutScaling=2^0
  Motor 2 : Outport  Port=2  OutDataType=sfix(16)  OutScaling=2^0
  Motor 3 : Outport  Port=3  OutDataType=sfix(16)  OutScaling=2^0
  Motor 4 : Outport  Port=4  OutDataType=sfix(16)  OutScaling=2^0
  wires:
  Motor Noise/1 -> Motor 1/1
  Motor Noise1/1 -> Motor 2/1
  Motor Noise2/1 -> Motor 3/1
  Motor Noise3/1 -> Motor 4/1

== system harness/Subsystem/Aerodynamic Effects/Moments/CrossProduct(AXB) ==
  A : Inport  OutDataType=sfix(16)  OutScaling=2^0
  B : Inport  Port=2  OutDataType=sfix(16)  OutScaling=2^0
  Fcn : Fcn  Expr=u[2]*u[6]-u[3]*u[5]
  Fcn1 : Fcn  Expr=u[3]*u[4]-u[1]*u[6]
  Fcn2 : Fcn  Expr=u[1]*u[5]-u[2]*u[4]
  Mux : Mux  Inputs=2
  Mux1 : Mux  Inputs=3
  Out : Outport  OutDataType=sfix(16)  OutScaling=2^0
  wires:
  A/1 -> Mux/1
  B/1 -> Mux/2
  Mux/1 -> Fcn/1, Fcn1/1, Fcn2/1
  Fcn/1 -> Mux1/1
  Fcn1/1 -> Mux1/2
  Fcn2/1 -> Mux1/3
  Mux1/1 -> Out/1

== system harness/Subsystem/Aerodynamic Effects/Moments/CrossProduct(AXB)1 ==
  A : Inport  OutDataType=sfix(16)  OutScaling=2^0
  B : Inport  Port=2  OutDataType=sfix(16)  OutScaling=2^0
  Fcn : Fcn  Expr=u[2]*u[6]-u[3]*u[5]
  Fcn1 : Fcn  Expr=u[3]*u[4]-u[1]*u[6]
  Fcn2 : Fcn  Expr=u[1]*u[5]-u[2]*u[4]
  Mux : Mux  Inputs=2
  Mux1 : Mux  Inputs=3
  Out : Outport  OutDataType=sfix(16)  OutScaling=2^0
  wires:
  Mux1/1 -> Out/1
  Fcn2/1 -> Mux1/3
  Fcn1/1 -> Mux1/2
  Fcn/1 -> Mux1/1
  Mux/1 -> Fcn2/1, Fcn1/1, Fcn/1
  B/1 -> Mux/2
  A/1 -> Mux/1

== system harness/Subsystem/Aerodynamic Effects/Moments/CrossProduct(AXB)2 ==
  A : Inport  OutDataType=sfix(16)  OutScaling=2^0
  B : Inport  Port=2  OutDataType=sfix(16)  OutScaling=2^0
  Fcn : Fcn  Expr=u[2]*u[6]-u[3]*u[5]
  Fcn1 : Fcn  Expr=u[3]*u[4]-u[1]*u[6]
  Fcn2 : Fcn  Expr=u[1]*u[5]-u[2]*u[4]
  Mux : Mux  Inputs=2
  Mux1 : Mux  Inputs=3
  Out : Outport  OutDataType=sfix(16)  OutScaling=2^0
  wires:
  A/1 -> Mux/1
  B/1 -> Mux/2
  Mux/1 -> Fcn/1, Fcn1/1, Fcn2/1
  Fcn/1 -> Mux1/1
  Fcn1/1 -> Mux1/2
  Fcn2/1 -> Mux1/3
  Mux1/1 -> Out/1

== system harness/Subsystem/Aerodynamic Effects/Moments/CrossProduct(AXB)3 ==
  A : Inport  OutDataType=sfix(16)  OutScaling=2^0
  B : Inport  Port=2  OutDataType=sfix(16)  OutScaling=2^0
  Fcn : Fcn  Expr=u[2]*u[6]-u[3]*u[5]
  Fcn1 : Fcn  Expr=u[3]*u[4]-u[1]*u[6]
  Fcn2 : Fcn  Expr=u[1]*u[5]-u[2]*u[4]
  Mux : Mux  Inputs=2
  Mux1 : Mux  Inputs=3
  Out : Outport  OutDataType=sfix(16)  OutScaling=2^0
  wires:
  Mux1/1 -> Out/1
  Fcn2/1 -> Mux1/3
  Fcn1/1 -> Mux1/2
  Fcn/1 -> Mux1/1
  Mux/1 -> Fcn2/1, Fcn1/1, Fcn/1
  B/1 -> Mux/2
  A/1 -> Mux/1

== system harness/Subsystem/Aerodynamic Effects/Moments/Motor Thrust to Torques ==
  Thrusts : Inport  OutDataType=sfix(16)  OutScaling=2^0
  Demux : Demux
  Gain1 : Gain  Gain=K_torque  ParameterDataType=sfix(16)  ParameterScaling=2^0  OutDataType=sfix(16)  OutScaling=2^0
  torque 1 : Outport  OutDataType=sfix(16)  OutScaling=2^0
  torque 2 : Outport  Port=2  OutDataType=sfix(16)  OutScaling=2^0
  torque 3 : Outport  Port=3  OutDataType=sfix(16)  OutScaling=2^0
  torque 4 : Outport  Port=4  OutDataType=sfix(16)  OutScaling=2^0
  wires:
  Thrusts/1 -> Gain1/1
  Gain1/1 -> Demux/1
  Demux/1 -> torque 1/1
  Demux/2 -> torque 2/1
  Demux/3 -> torque 3/1
  Demux/4 -> torque 4/1

== system harness/Subsystem/Aerodynamic Effects/Vertical Effect Dynamics/Motor 1 Vertical Effect Dynamics ==
  Thrust Command : Inport  OutDataType=sfix(16)  OutScaling=2^0
  V (body) : Inport  Port=2  OutDataType=sfix(16)  OutScaling=2^0
  Abs : Abs
  Constant : Constant  OutDataType=sfix(16)  OutScaling=2^0
  Demux : Demux  Outputs=3
  Divide : Product  Inputs=*/  OutDataType=sfix(16)  OutScaling=2^-10
  Dot Product : simulink/Math Operations/Dot Product  InputSameDT=on  OutDataType=sfix(16)  OutScaling=2^-10  DoSatur=off
  Math Function : Math  Operator=sqrt  OutDataType=sfix(16)  OutScaling=2^0  SaturateOnIntegerOverflow=on
  Saturation : Saturate  UpperLimit=500000  LowerLimit=0.0000000001
  Switch : Switch  Threshold=1.2
  T : Terminator
  T1 : Terminator
  TM1 : Scope
      settings: YMin=-1  YMax=11  SaveName=ScopeData18
  Trigonometric Function : Trigonometry  Operator=asin
  Unary Minus : simulink/Math Operations/Unary Minus  DoSatur=off
  alpha : Scope
      settings: YMin=-1.25  YMax=1.75  SaveName=ScopeData17
  v_h : Scope
      settings: YMin=-1  YMax=11  SaveName=ScopeData15
  "v_h " : Fcn  Expr=sqrt(u/(2*rho*A))
  v_i Lookup Table (n-D) : Lookup_n-D  NumberOfTableDimensions=3  BreakpointsForDimension1=Alpha  BreakpointsForDimension2=Vinf  BreakpointsForDimension3=Vh  BeginIndexSearchUsingPreviousIndexResult=on  Table=ToverTh  InterpMethod=Cubic spline
  v_inf{,1..3} (4 alike) : Scope
      v_inf settings: YMin=-1  YMax=11  SaveName=ScopeData16
      v_inf1 settings: TimeRange=20  YMin=-0.5  YMax=0.6  SaveName=ScopeData13
      v_inf2 settings: YMin=-1  YMax=1  SaveName=ScopeData19
      v_inf3 settings: TimeRange=20  YMin=0  YMax=5.5  SaveName=ScopeData20
  Thrust Multiplier : Outport  OutDataType=sfix(16)  OutScaling=2^0
  wires:
  Thrust Command/1 -> "v_h "/1
  V (body)/1 -> Dot Product/1, Dot Product/2, Demux/1
  "v_h "/1 -> v_h/1, v_i Lookup Table (n-D)/3
  Dot Product/1 -> Math Function/1
  Math Function/1 -> v_inf/1, v_i Lookup Table (n-D)/2, Saturation/1  "v_inf"
  Demux/1 -> T/1
  Demux/2 -> T1/1
  Divide/1 -> Trigonometric Function/1, v_inf2/1
  Trigonometric Function/1 -> alpha/1, Abs/1, v_i Lookup Table (n-D)/1  "alpha"
  Switch/1 -> Thrust Multiplier/1
  v_i Lookup Table (n-D)/1 -> Switch/3, TM1/1
  Constant/1 -> Switch/1
  Abs/1 -> Switch/2
  Unary Minus/1 -> Divide/1, v_inf1/1
  Demux/3 -> Unary Minus/1
  Saturation/1 -> Divide/2, v_inf3/1

== system harness/Subsystem/Aerodynamic Effects/Vertical Effect Dynamics/Motor 2 Vertical Effect Dynamics ==
  Thrust Command : Inport  OutDataType=sfix(16)  OutScaling=2^0
  V (body) : Inport  Port=2  OutDataType=sfix(16)  OutScaling=2^0
  Abs : Abs
  Constant : Constant  OutDataType=sfix(16)  OutScaling=2^0
  Demux : Demux  Outputs=3
  Divide : Product  Inputs=*/  OutDataType=sfix(16)  OutScaling=2^-10
  Dot Product : simulink/Math Operations/Dot Product  InputSameDT=on  OutDataType=sfix(16)  OutScaling=2^-10  DoSatur=off
  Math Function : Math  Operator=sqrt  OutDataType=sfix(16)  OutScaling=2^0  SaturateOnIntegerOverflow=on
  Saturation : Saturate  UpperLimit=500000  LowerLimit=0.00001
  Switch : Switch  Threshold=0.5
  T : Terminator
  T1 : Terminator
  TM1 : Scope
      settings: YMin=-1  YMax=11  SaveName=ScopeData18
  Trigonometric Function : Trigonometry  Operator=asin
  Unary Minus : simulink/Math Operations/Unary Minus  DoSatur=off
  alpha : Scope
      settings: YMin=0  YMax=1.75  SaveName=ScopeData17
  v_h : Scope
      settings: YMin=-1  YMax=11  SaveName=ScopeData15
  "v_h " : Fcn  Expr=sqrt(u/(2*rho*A))
  v_i Lookup Table (n-D) : Lookup_n-D  NumberOfTableDimensions=3  BreakpointsForDimension1=Alpha  BreakpointsForDimension2=Vinf  BreakpointsForDimension3=Vh  BeginIndexSearchUsingPreviousIndexResult=on  Table=ToverTh  InterpMethod=Cubic spline
  v_inf : Scope
      settings: YMin=-1  YMax=11  SaveName=ScopeData16
  Thrust Multiplier : Outport  OutDataType=sfix(16)  OutScaling=2^0
  wires:
  Thrust Command/1 -> "v_h "/1
  V (body)/1 -> Dot Product/1, Dot Product/2, Demux/1
  "v_h "/1 -> v_h/1, v_i Lookup Table (n-D)/3
  Dot Product/1 -> Math Function/1
  Math Function/1 -> v_inf/1, v_i Lookup Table (n-D)/2, Saturation/1  "v_inf"
  Demux/1 -> T/1
  Demux/2 -> T1/1
  Divide/1 -> Trigonometric Function/1
  Trigonometric Function/1 -> alpha/1, Abs/1, v_i Lookup Table (n-D)/1  "alpha"
  Switch/1 -> Thrust Multiplier/1
  v_i Lookup Table (n-D)/1 -> Switch/3, TM1/1
  Constant/1 -> Switch/1
  Abs/1 -> Switch/2
  Unary Minus/1 -> Divide/1
  Demux/3 -> Unary Minus/1
  Saturation/1 -> Divide/2

== system harness/Subsystem/Aerodynamic Effects/Vertical Effect Dynamics/Motor 3 Vertical Effect Dynamics ==
  Thrust Command : Inport  OutDataType=sfix(16)  OutScaling=2^0
  V (body) : Inport  Port=2  OutDataType=sfix(16)  OutScaling=2^0
  Abs : Abs
  Constant : Constant  OutDataType=sfix(16)  OutScaling=2^0
  Demux : Demux  Outputs=3
  Divide : Product  Inputs=*/  OutDataType=sfix(16)  OutScaling=2^-10
  Dot Product : simulink/Math Operations/Dot Product  InputSameDT=on  OutDataType=sfix(16)  OutScaling=2^-10  DoSatur=off
  Math Function : Math  Operator=sqrt  OutDataType=sfix(16)  OutScaling=2^0  SaturateOnIntegerOverflow=on
  Saturation : Saturate  UpperLimit=500000  LowerLimit=0.00001
  Switch : Switch  Threshold=0.5
  T : Terminator
  T1 : Terminator
  TM1 : Scope
      settings: YMin=-1  YMax=11  SaveName=ScopeData18
  Trigonometric Function : Trigonometry  Operator=asin
  Unary Minus : simulink/Math Operations/Unary Minus  DoSatur=off
  alpha : Scope
      settings: YMin=0  YMax=1.75  SaveName=ScopeData17
  v_h : Scope
      settings: YMin=-1  YMax=11  SaveName=ScopeData15
  "v_h " : Fcn  Expr=sqrt(u/(2*rho*A))
  v_i Lookup Table (n-D) : Lookup_n-D  NumberOfTableDimensions=3  BreakpointsForDimension1=Alpha  BreakpointsForDimension2=Vinf  BreakpointsForDimension3=Vh  BeginIndexSearchUsingPreviousIndexResult=on  Table=ToverTh  InterpMethod=Cubic spline
  v_inf : Scope
      settings: YMin=-1  YMax=11  SaveName=ScopeData16
  Thrust Multiplier : Outport  OutDataType=sfix(16)  OutScaling=2^0
  wires:
  Thrust Command/1 -> "v_h "/1
  V (body)/1 -> Dot Product/1, Dot Product/2, Demux/1
  "v_h "/1 -> v_h/1, v_i Lookup Table (n-D)/3
  Dot Product/1 -> Math Function/1
  Math Function/1 -> v_inf/1, v_i Lookup Table (n-D)/2, Saturation/1  "v_inf"
  Demux/1 -> T/1
  Demux/2 -> T1/1
  Divide/1 -> Trigonometric Function/1
  Trigonometric Function/1 -> alpha/1, Abs/1, v_i Lookup Table (n-D)/1  "alpha"
  Switch/1 -> Thrust Multiplier/1
  v_i Lookup Table (n-D)/1 -> Switch/3, TM1/1
  Constant/1 -> Switch/1
  Abs/1 -> Switch/2
  Unary Minus/1 -> Divide/1
  Demux/3 -> Unary Minus/1
  Saturation/1 -> Divide/2

== system harness/Subsystem/Aerodynamic Effects/Vertical Effect Dynamics/Motor 4 Vertical Effect Dynamics ==
  Thrust Command : Inport  OutDataType=sfix(16)  OutScaling=2^0
  V (body) : Inport  Port=2  OutDataType=sfix(16)  OutScaling=2^0
  Abs : Abs
  Constant : Constant  OutDataType=sfix(16)  OutScaling=2^0
  Demux : Demux  Outputs=3
  Divide : Product  Inputs=*/  OutDataType=sfix(16)  OutScaling=2^-10
  Dot Product : simulink/Math Operations/Dot Product  InputSameDT=on  OutDataType=sfix(16)  OutScaling=2^-10  DoSatur=off
  Math Function : Math  Operator=sqrt  OutDataType=sfix(16)  OutScaling=2^0  SaturateOnIntegerOverflow=on
  Saturation : Saturate  UpperLimit=500000  LowerLimit=0.00001
  Switch : Switch  Threshold=0.5
  T : Terminator
  T1 : Terminator
  TM1 : Scope
      settings: YMin=-1  YMax=11  SaveName=ScopeData18
  Trigonometric Function : Trigonometry  Operator=asin
  Unary Minus : simulink/Math Operations/Unary Minus  DoSatur=off
  alpha : Scope
      settings: YMin=0  YMax=1.75  SaveName=ScopeData17
  v_h : Scope
      settings: YMin=-1  YMax=11  SaveName=ScopeData15
  "v_h " : Fcn  Expr=sqrt(u/(2*rho*A))
  v_i Lookup Table (n-D) : Lookup_n-D  NumberOfTableDimensions=3  BreakpointsForDimension1=Alpha  BreakpointsForDimension2=Vinf  BreakpointsForDimension3=Vh  BeginIndexSearchUsingPreviousIndexResult=on  Table=ToverTh  InterpMethod=Cubic spline
  v_inf : Scope
      settings: YMin=-1  YMax=11  SaveName=ScopeData16
  Thrust Multiplier : Outport  OutDataType=sfix(16)  OutScaling=2^0
  wires:
  Thrust Command/1 -> "v_h "/1
  V (body)/1 -> Dot Product/1, Dot Product/2, Demux/1
  "v_h "/1 -> v_h/1, v_i Lookup Table (n-D)/3
  Dot Product/1 -> Math Function/1
  Math Function/1 -> v_inf/1, v_i Lookup Table (n-D)/2, Saturation/1  "v_inf"
  Demux/1 -> T/1
  Demux/2 -> T1/1
  Divide/1 -> Trigonometric Function/1
  Trigonometric Function/1 -> alpha/1, Abs/1, v_i Lookup Table (n-D)/1  "alpha"
  Switch/1 -> Thrust Multiplier/1
  v_i Lookup Table (n-D)/1 -> Switch/3, TM1/1
  Constant/1 -> Switch/1
  Abs/1 -> Switch/2
  Unary Minus/1 -> Divide/1
  Demux/3 -> Unary Minus/1
  Saturation/1 -> Divide/2

== system harness/Subsystem1/Aerodynamic Effects/Moments/CrossProduct(AXB) ==
  A : Inport  OutDataType=sfix(16)  OutScaling=2^0
  B : Inport  Port=2  OutDataType=sfix(16)  OutScaling=2^0
  Fcn : Fcn  Expr=u[2]*u[6]-u[3]*u[5]
  Fcn1 : Fcn  Expr=u[3]*u[4]-u[1]*u[6]
  Fcn2 : Fcn  Expr=u[1]*u[5]-u[2]*u[4]
  Mux : Mux  Inputs=2
  Mux1 : Mux  Inputs=3
  Out : Outport  OutDataType=sfix(16)  OutScaling=2^0
  wires:
  A/1 -> Mux/1
  B/1 -> Mux/2
  Mux/1 -> Fcn/1, Fcn1/1, Fcn2/1
  Fcn/1 -> Mux1/1
  Fcn1/1 -> Mux1/2
  Fcn2/1 -> Mux1/3
  Mux1/1 -> Out/1

== system harness/Subsystem1/Aerodynamic Effects/Moments/CrossProduct(AXB)1 ==
  A : Inport  OutDataType=sfix(16)  OutScaling=2^0
  B : Inport  Port=2  OutDataType=sfix(16)  OutScaling=2^0
  Fcn : Fcn  Expr=u[2]*u[6]-u[3]*u[5]
  Fcn1 : Fcn  Expr=u[3]*u[4]-u[1]*u[6]
  Fcn2 : Fcn  Expr=u[1]*u[5]-u[2]*u[4]
  Mux : Mux  Inputs=2
  Mux1 : Mux  Inputs=3
  Out : Outport  OutDataType=sfix(16)  OutScaling=2^0
  wires:
  Mux1/1 -> Out/1
  Fcn2/1 -> Mux1/3
  Fcn1/1 -> Mux1/2
  Fcn/1 -> Mux1/1
  Mux/1 -> Fcn2/1, Fcn1/1, Fcn/1
  B/1 -> Mux/2
  A/1 -> Mux/1

== system harness/Subsystem1/Aerodynamic Effects/Moments/CrossProduct(AXB)2 ==
  A : Inport  OutDataType=sfix(16)  OutScaling=2^0
  B : Inport  Port=2  OutDataType=sfix(16)  OutScaling=2^0
  Fcn : Fcn  Expr=u[2]*u[6]-u[3]*u[5]
  Fcn1 : Fcn  Expr=u[3]*u[4]-u[1]*u[6]
  Fcn2 : Fcn  Expr=u[1]*u[5]-u[2]*u[4]
  Mux : Mux  Inputs=2
  Mux1 : Mux  Inputs=3
  Out : Outport  OutDataType=sfix(16)  OutScaling=2^0
  wires:
  A/1 -> Mux/1
  B/1 -> Mux/2
  Mux/1 -> Fcn/1, Fcn1/1, Fcn2/1
  Fcn/1 -> Mux1/1
  Fcn1/1 -> Mux1/2
  Fcn2/1 -> Mux1/3
  Mux1/1 -> Out/1

== system harness/Subsystem1/Aerodynamic Effects/Moments/CrossProduct(AXB)3 ==
  A : Inport  OutDataType=sfix(16)  OutScaling=2^0
  B : Inport  Port=2  OutDataType=sfix(16)  OutScaling=2^0
  Fcn : Fcn  Expr=u[2]*u[6]-u[3]*u[5]
  Fcn1 : Fcn  Expr=u[3]*u[4]-u[1]*u[6]
  Fcn2 : Fcn  Expr=u[1]*u[5]-u[2]*u[4]
  Mux : Mux  Inputs=2
  Mux1 : Mux  Inputs=3
  Out : Outport  OutDataType=sfix(16)  OutScaling=2^0
  wires:
  Mux1/1 -> Out/1
  Fcn2/1 -> Mux1/3
  Fcn1/1 -> Mux1/2
  Fcn/1 -> Mux1/1
  Mux/1 -> Fcn2/1, Fcn1/1, Fcn/1
  B/1 -> Mux/2
  A/1 -> Mux/1

== system harness/Subsystem1/Aerodynamic Effects/Moments/Motor Thrust to Torques ==
  Thrusts : Inport  OutDataType=sfix(16)  OutScaling=2^0
  Demux : Demux
  Gain1 : Gain  Gain=K_torque  ParameterDataType=sfix(16)  ParameterScaling=2^0  OutDataType=sfix(16)  OutScaling=2^0
  torque 1 : Outport  OutDataType=sfix(16)  OutScaling=2^0
  torque 2 : Outport  Port=2  OutDataType=sfix(16)  OutScaling=2^0
  torque 3 : Outport  Port=3  OutDataType=sfix(16)  OutScaling=2^0
  torque 4 : Outport  Port=4  OutDataType=sfix(16)  OutScaling=2^0
  wires:
  Thrusts/1 -> Gain1/1
  Gain1/1 -> Demux/1
  Demux/1 -> torque 1/1
  Demux/2 -> torque 2/1
  Demux/3 -> torque 3/1
  Demux/4 -> torque 4/1

== system harness/Subsystem1/Aerodynamic Effects/Vertical Effect Dynamics/Motor 1 Vertical Effect Dynamics ==
  Thrust Command : Inport  OutDataType=sfix(16)  OutScaling=2^0
  V (body) : Inport  Port=2  OutDataType=sfix(16)  OutScaling=2^0
  Abs : Abs
  Constant : Constant  OutDataType=sfix(16)  OutScaling=2^0
  Demux : Demux  Outputs=3
  Divide : Product  Inputs=*/  OutDataType=sfix(16)  OutScaling=2^-10
  Dot Product : simulink/Math Operations/Dot Product  InputSameDT=on  OutDataType=sfix(16)  OutScaling=2^-10  DoSatur=off
  Math Function : Math  Operator=sqrt  OutDataType=sfix(16)  OutScaling=2^0  SaturateOnIntegerOverflow=on
  Saturation : Saturate  UpperLimit=500000  LowerLimit=0.0000000001
  Switch : Switch  Threshold=1.2
  T : Terminator
  T1 : Terminator
  TM1 : Scope
      settings: YMin=-1  YMax=11  SaveName=ScopeData18
  Trigonometric Function : Trigonometry  Operator=asin
  Unary Minus : simulink/Math Operations/Unary Minus  DoSatur=off
  alpha : Scope
      settings: YMin=-1.25  YMax=1.75  SaveName=ScopeData17
  v_h : Scope
      settings: YMin=-1  YMax=11  SaveName=ScopeData15
  "v_h " : Fcn  Expr=sqrt(u/(2*rho*A))
  v_i Lookup Table (n-D) : Lookup_n-D  NumberOfTableDimensions=3  BreakpointsForDimension1=Alpha  BreakpointsForDimension2=Vinf  BreakpointsForDimension3=Vh  BeginIndexSearchUsingPreviousIndexResult=on  Table=ToverTh  InterpMethod=Cubic spline
  v_inf{,1..3} (4 alike) : Scope
      v_inf settings: YMin=-1  YMax=11  SaveName=ScopeData16
      v_inf1 settings: TimeRange=20  YMin=-0.5  YMax=0.6  SaveName=ScopeData13
      v_inf2 settings: YMin=-1  YMax=1  SaveName=ScopeData19
      v_inf3 settings: TimeRange=20  YMin=0  YMax=5.5  SaveName=ScopeData20
  Thrust Multiplier : Outport  OutDataType=sfix(16)  OutScaling=2^0
  wires:
  Thrust Command/1 -> "v_h "/1
  V (body)/1 -> Dot Product/1, Dot Product/2, Demux/1
  "v_h "/1 -> v_h/1, v_i Lookup Table (n-D)/3
  Dot Product/1 -> Math Function/1
  Math Function/1 -> v_inf/1, v_i Lookup Table (n-D)/2, Saturation/1  "v_inf"
  Demux/1 -> T/1
  Demux/2 -> T1/1
  Divide/1 -> Trigonometric Function/1, v_inf2/1
  Trigonometric Function/1 -> alpha/1, Abs/1, v_i Lookup Table (n-D)/1  "alpha"
  Switch/1 -> Thrust Multiplier/1
  v_i Lookup Table (n-D)/1 -> Switch/3, TM1/1
  Constant/1 -> Switch/1
  Abs/1 -> Switch/2
  Unary Minus/1 -> Divide/1, v_inf1/1
  Demux/3 -> Unary Minus/1
  Saturation/1 -> Divide/2, v_inf3/1

== system harness/Subsystem1/Aerodynamic Effects/Vertical Effect Dynamics/Motor 2 Vertical Effect Dynamics ==
  Thrust Command : Inport  OutDataType=sfix(16)  OutScaling=2^0
  V (body) : Inport  Port=2  OutDataType=sfix(16)  OutScaling=2^0
  Abs : Abs
  Constant : Constant  OutDataType=sfix(16)  OutScaling=2^0
  Demux : Demux  Outputs=3
  Divide : Product  Inputs=*/  OutDataType=sfix(16)  OutScaling=2^-10
  Dot Product : simulink/Math Operations/Dot Product  InputSameDT=on  OutDataType=sfix(16)  OutScaling=2^-10  DoSatur=off
  Math Function : Math  Operator=sqrt  OutDataType=sfix(16)  OutScaling=2^0  SaturateOnIntegerOverflow=on
  Saturation : Saturate  UpperLimit=500000  LowerLimit=0.00001
  Switch : Switch  Threshold=0.5
  T : Terminator
  T1 : Terminator
  TM1 : Scope
      settings: YMin=-1  YMax=11  SaveName=ScopeData18
  Trigonometric Function : Trigonometry  Operator=asin
  Unary Minus : simulink/Math Operations/Unary Minus  DoSatur=off
  alpha : Scope
      settings: YMin=0  YMax=1.75  SaveName=ScopeData17
  v_h : Scope
      settings: YMin=-1  YMax=11  SaveName=ScopeData15
  "v_h " : Fcn  Expr=sqrt(u/(2*rho*A))
  v_i Lookup Table (n-D) : Lookup_n-D  NumberOfTableDimensions=3  BreakpointsForDimension1=Alpha  BreakpointsForDimension2=Vinf  BreakpointsForDimension3=Vh  BeginIndexSearchUsingPreviousIndexResult=on  Table=ToverTh  InterpMethod=Cubic spline
  v_inf : Scope
      settings: YMin=-1  YMax=11  SaveName=ScopeData16
  Thrust Multiplier : Outport  OutDataType=sfix(16)  OutScaling=2^0
  wires:
  Thrust Command/1 -> "v_h "/1
  V (body)/1 -> Dot Product/1, Dot Product/2, Demux/1
  "v_h "/1 -> v_h/1, v_i Lookup Table (n-D)/3
  Dot Product/1 -> Math Function/1
  Math Function/1 -> v_inf/1, v_i Lookup Table (n-D)/2, Saturation/1  "v_inf"
  Demux/1 -> T/1
  Demux/2 -> T1/1
  Divide/1 -> Trigonometric Function/1
  Trigonometric Function/1 -> alpha/1, Abs/1, v_i Lookup Table (n-D)/1  "alpha"
  Switch/1 -> Thrust Multiplier/1
  v_i Lookup Table (n-D)/1 -> Switch/3, TM1/1
  Constant/1 -> Switch/1
  Abs/1 -> Switch/2
  Unary Minus/1 -> Divide/1
  Demux/3 -> Unary Minus/1
  Saturation/1 -> Divide/2

== system harness/Subsystem1/Aerodynamic Effects/Vertical Effect Dynamics/Motor 3 Vertical Effect Dynamics ==
  Thrust Command : Inport  OutDataType=sfix(16)  OutScaling=2^0
  V (body) : Inport  Port=2  OutDataType=sfix(16)  OutScaling=2^0
  Abs : Abs
  Constant : Constant  OutDataType=sfix(16)  OutScaling=2^0
  Demux : Demux  Outputs=3
  Divide : Product  Inputs=*/  OutDataType=sfix(16)  OutScaling=2^-10
  Dot Product : simulink/Math Operations/Dot Product  InputSameDT=on  OutDataType=sfix(16)  OutScaling=2^-10  DoSatur=off
  Math Function : Math  Operator=sqrt  OutDataType=sfix(16)  OutScaling=2^0  SaturateOnIntegerOverflow=on
  Saturation : Saturate  UpperLimit=500000  LowerLimit=0.00001
  Switch : Switch  Threshold=0.5
  T : Terminator
  T1 : Terminator
  TM1 : Scope
      settings: YMin=-1  YMax=11  SaveName=ScopeData18
  Trigonometric Function : Trigonometry  Operator=asin
  Unary Minus : simulink/Math Operations/Unary Minus  DoSatur=off
  alpha : Scope
      settings: YMin=0  YMax=1.75  SaveName=ScopeData17
  v_h : Scope
      settings: YMin=-1  YMax=11  SaveName=ScopeData15
  "v_h " : Fcn  Expr=sqrt(u/(2*rho*A))
  v_i Lookup Table (n-D) : Lookup_n-D  NumberOfTableDimensions=3  BreakpointsForDimension1=Alpha  BreakpointsForDimension2=Vinf  BreakpointsForDimension3=Vh  BeginIndexSearchUsingPreviousIndexResult=on  Table=ToverTh  InterpMethod=Cubic spline
  v_inf : Scope
      settings: YMin=-1  YMax=11  SaveName=ScopeData16
  Thrust Multiplier : Outport  OutDataType=sfix(16)  OutScaling=2^0
  wires:
  Thrust Command/1 -> "v_h "/1
  V (body)/1 -> Dot Product/1, Dot Product/2, Demux/1
  "v_h "/1 -> v_h/1, v_i Lookup Table (n-D)/3
  Dot Product/1 -> Math Function/1
  Math Function/1 -> v_inf/1, v_i Lookup Table (n-D)/2, Saturation/1  "v_inf"
  Demux/1 -> T/1
  Demux/2 -> T1/1
  Divide/1 -> Trigonometric Function/1
  Trigonometric Function/1 -> alpha/1, Abs/1, v_i Lookup Table (n-D)/1  "alpha"
  Switch/1 -> Thrust Multiplier/1
  v_i Lookup Table (n-D)/1 -> Switch/3, TM1/1
  Constant/1 -> Switch/1
  Abs/1 -> Switch/2
  Unary Minus/1 -> Divide/1
  Demux/3 -> Unary Minus/1
  Saturation/1 -> Divide/2
